simulink model "SMART_GRID_EV_as_an_Ancillary"  (R2021a)
settings: Solver=ode23tb  StartTime=0.0  StopTime=0.3  MaxStep=1e-5  RelTol=1e-3
undefined symbols (not defined in the file): DiscIntNeverNeededParam, Ion, Lithium
libraries: powerlib_extras x6, spsThreePhaseSeriesRLCBranchLib x4, spsThreePhaseVIMeasurementLib x3, spsGroundLib x2, spsBatteryLib x1, simulink x1, spsUniversalBridgeLib x1, spsThreePhaseSourceLib x1, spsThreePhaseBreakerLib x1, spspowerguiLib x1
settings Model: Creator=mo saf  LastModifiedBy=raiaj
settings SolverCC: ZeroCrossControl=DisableAll  SolverResetMethod=Robust

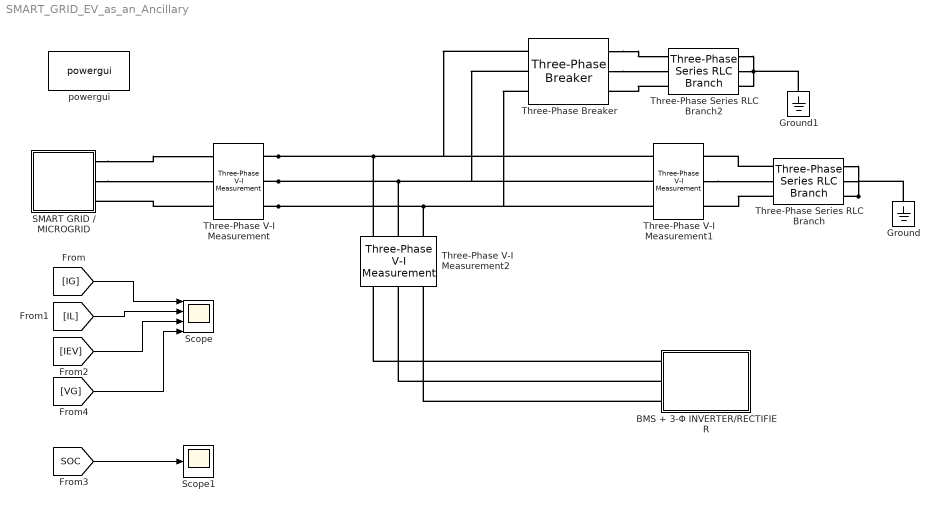
== system SMART_GRID_EV_as_an_Ancillary ==
  BMS + 3-Φ INVERTER/RECTIFIER : Subsystem
  Ground : spsGroundLib/Ground  LConnTagsString=a
  Ground1 : spsGroundLib/Ground  LConnTagsString=a
  SMART GRID / MICROGRID : Subsystem
  Scope : Scope  NumInputPorts=4
  Scope1 : Scope
  Three-Phase Series RLC Branch : spsThreePhaseSeriesRLCBranchLib/Three-Phase Series RLC Branch  LConnTagsString=A|B|C  RConnTagsString=A|B|C  BranchType=R  Resistance=20  Inductance=1e-3  Capacitance=1e-6  Measurements=None
  Three-Phase Series RLC Branch2 : spsThreePhaseSeriesRLCBranchLib/Three-Phase Series RLC Branch  LConnTagsString=A|B|C  RConnTagsString=A|B|C  BranchType=R  Resistance=6  Inductance=1e-3  Capacitance=1e-6  Measurements=None
  Three-Phase V-I Measurement : spsThreePhaseVIMeasurementLib/Three-Phase V-I Measurement  VoltageMeasurement=phase-to-ground  SetLabelV=on  LabelV=VG  Vpu=off  VpuLL=off  CurrentMeasurement=yes  SetLabelI=on  LabelI=IG  Ipu=off  Pbase=100e6  Vbase=500e3  OutputType=Complex  PhasorSimulation=off  PSBequivalent=0
  Three-Phase V-I Measurement1 : spsThreePhaseVIMeasurementLib/Three-Phase V-I Measurement  VoltageMeasurement=phase-to-ground  SetLabelV=on  LabelV=VL  Vpu=off  VpuLL=off  CurrentMeasurement=yes  SetLabelI=on  LabelI=IL  Ipu=off  Pbase=100e6  Vbase=500e3  OutputType=Complex  PhasorSimulation=off  PSBequivalent=0
  Three-Phase V-I Measurement2 : spsThreePhaseVIMeasurementLib/Three-Phase V-I Measurement  VoltageMeasurement=phase-to-ground  SetLabelV=on  LabelV=VEV  Vpu=off  VpuLL=off  CurrentMeasurement=yes  SetLabelI=on  LabelI=IEV  Ipu=off  Pbase=100e6  Vbase=500e3  OutputType=Complex  PhasorSimulation=off  PSBequivalent=0
  Three-Phase Breaker : spsThreePhaseBreakerLib/Three-Phase Breaker  InitialState=open  SwitchA=on  SwitchB=on  SwitchC=on  SwitchTimes=[0.1 9]  External=off  BreakerResistance=0.01  SnubberResistance=1e6  SnubberCapacitance=inf  Measurements=None
  powergui : spspowerguiLib/powergui  Priority=1  SimulationMode=Continuous  SampleTime=50e-6  frequency=60  Iterations=50  frequencyindice=50  Pbase=100e6  ErrMax=1e-4  UnitsV=kV  UnitsW=MW  buscounter=0  FunctionMessages=off  echomessages=off  EnableUseOfTLC=off  CurrentSourceSwitches=off  DisableSnubberDevices=off  DisableRonSwitches=off  DisableVfSwitches=off  DisplayEquations=off  AutomaticDiscreteSolvers=off  SolverType=Tustin/Backward Euler (TBE)  Interpol=off  ExternalGateDelay=off  methode=off  Ts=100  x0status=blocks  SPID=on  SwTol=0  HookPort=off  NonlinearTolerance=1e-4  nMaxIteration=100  ContinueOnMaxIteration=off  RestoreLinks=warning  ResistiveCurrentMeasurement=off  Frange=[0:2:500]  Ylog=off  Xlog=on  ShowGrid=off  save=off  variable=ZData  structure=0  ZoomFFT=off  StartTime=0.0  cycles=1  DisplayStyle=1  fundamental=60  FreqAxis=off  MaxFrequency=1000  frequencyindicesteady=1  RmsSteady=1  display=off
  wires:
  [IG] -> Scope/1
  [IEV] -> Scope/3
  [IL] -> Scope/2
  [VG] -> Scope/4
  [SOC] -> Scope1/1
  connections:
  Three-Phase V-I Measurement/RConn2 -- Three-Phase V-I Measurement2/RConn2 -- Three-Phase V-I Measurement1/LConn2 -- Three-Phase Breaker/LConn2
  Three-Phase V-I Measurement/RConn3 -- Three-Phase V-I Measurement2/RConn3 -- Three-Phase V-I Measurement1/LConn3 -- Three-Phase Breaker/LConn3
  Three-Phase Series RLC Branch2/RConn2 -- Ground1/LConn1 -- Three-Phase Series RLC Branch2/RConn1 -- Three-Phase Series RLC Branch2/RConn3
  Three-Phase Series RLC Branch/RConn3 -- Three-Phase Series RLC Branch/RConn1 -- Ground/LConn1 -- Three-Phase Series RLC Branch/RConn2
  Three-Phase V-I Measurement/RConn1 -- Three-Phase V-I Measurement1/LConn1 -- Three-Phase Breaker/LConn1 -- Three-Phase V-I Measurement2/RConn1
  Three-Phase Series RLC Branch/LConn1 -- Three-Phase V-I Measurement1/RConn1
  Three-Phase Series RLC Branch2/LConn3 -- Three-Phase Breaker/RConn3
  Three-Phase Series RLC Branch/LConn3 -- Three-Phase V-I Measurement1/RConn3
  Three-Phase V-I Measurement1/RConn2 -- Three-Phase Series RLC Branch/LConn2
  Three-Phase Breaker/RConn2 -- Three-Phase Series RLC Branch2/LConn2
  Three-Phase Breaker/RConn1 -- Three-Phase Series RLC Branch2/LConn1
  SMART GRID / MICROGRID/RConn1 -- Three-Phase V-I Measurement/LConn1
  SMART GRID / MICROGRID/RConn2 -- Three-Phase V-I Measurement/LConn2
  Three-Phase V-I Measurement/LConn3 -- SMART GRID / MICROGRID/RConn3
  BMS + 3-Φ INVERTER/RECTIFIER/LConn1 -- Three-Phase V-I Measurement2/LConn1
  BMS + 3-Φ INVERTER/RECTIFIER/LConn2 -- Three-Phase V-I Measurement2/LConn2
  BMS + 3-Φ INVERTER/RECTIFIER/LConn3 -- Three-Phase V-I Measurement2/LConn3

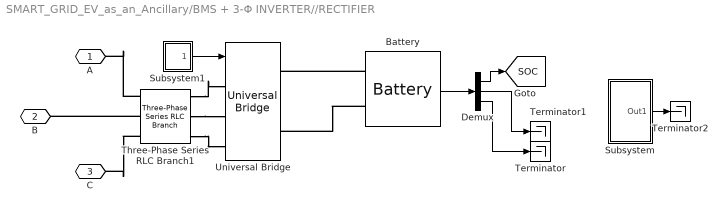
== system SMART_GRID_EV_as_an_Ancillary/BMS + 3-Φ INVERTER//RECTIFIER ==
  Battery : spsBatteryLib/Battery  BatType=Lithium-Ion  ShowTempParam=off  ThermalPreset=no  ShowAgeParam=off  NomV=700  NomQ=20  SOC=100  Batt_Tr=30  PresetModel=on  MaxQ=20  MinV=525  FullV=814.791  Dis_rate=8.6957  R=0.35  Normal_OP=18.087  expZone="[756.2701     0.9826087]"  current=[6.5 13 32.5]  Units=Time  Tci=20  NomT=20  T2=-30  MaxQ2=4.8  FullV2=7.1  Normal_OP2=5.655  expZone2="[6.58           1]"  Rca=0.6  ti=2000  Dp=0  Neq0=0  Tsim=1e6  Ta1=25  Qeol=5.4*0.9  Reol=0.013333*1.2  Char_age=[2.3478, 3]  Dis_age=[2.3478, 10]  N1=1500  N2=10500  N3=1000  N4=1400  Ta2=45  N5=950
  Demux : Demux  Outputs=3
  Subsystem : Subsystem
  Subsystem1 : Subsystem
  Terminator : Terminator
  Terminator1 : Terminator
  Terminator2 : Terminator
  Three-Phase Series RLC Branch1 : spsThreePhaseSeriesRLCBranchLib/Three-Phase Series RLC Branch  LConnTagsString=A|B|C  RConnTagsString=A|B|C  BranchType=L  Resistance=100  Inductance=2.5e-3  Capacitance=1e-6  Measurements=None
  Universal Bridge : spsUniversalBridgeLib/Universal Bridge  Arms=3  SnubberResistance=1e5  SnubberCapacitance=inf  Device=IGBT / Diodes  Ron=1e-3  Lon=0  ForwardVoltages="[  0  0  ]"  ForwardVoltage=0  GTOparameters=[ 10e-6 , 20e-6 ]  IGBTparameters=[ 1e-6 , 2e-6 ]  Measurements=None  Measurements_2=None  converterType=Rectifier
  A : PMIOPort  Side=Left
  B : PMIOPort  Port=2  Side=Left
  C : PMIOPort  Port=3  Side=Left
  tag scope: SOC=global
  wires:
  Battery/1 -> Demux/1
  Demux/2 -> Terminator1/1
  Demux/1 -> [SOC]
  Demux/3 -> Terminator/1
  Subsystem1/1(Out1) -> Universal Bridge/1
  Subsystem/1(Out1) -> Terminator2/1
  connections:
  Three-Phase Series RLC Branch1/RConn3 -- Universal Bridge/LConn3
  Battery/LConn2 -- Universal Bridge/RConn2
  Battery/LConn1 -- Universal Bridge/RConn1
  Three-Phase Series RLC Branch1/RConn2 -- Universal Bridge/LConn2
  Three-Phase Series RLC Branch1/RConn1 -- Universal Bridge/LConn1
  Three-Phase Series RLC Branch1/LConn3 -- C/RConn1
  Three-Phase Series RLC Branch1/LConn1 -- A/RConn1
  Three-Phase Series RLC Branch1/LConn2 -- B/RConn1

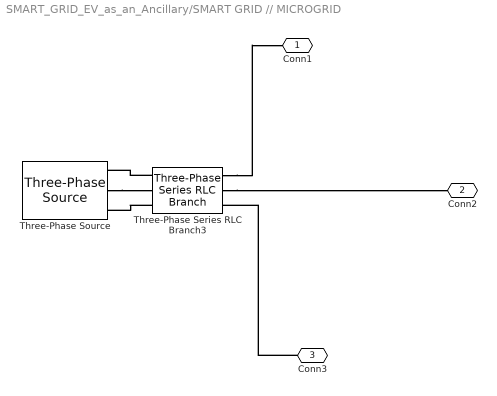
== system SMART_GRID_EV_as_an_Ancillary/SMART GRID // MICROGRID ==
  Three-Phase Series RLC Branch3 : spsThreePhaseSeriesRLCBranchLib/Three-Phase Series RLC Branch  LConnTagsString=A|B|C  RConnTagsString=A|B|C  BranchType=R  Resistance=0.1  Inductance=1e-3  Capacitance=1e-6  Measurements=None
  Three-Phase Source : spsThreePhaseSourceLib/Three-Phase Source  InternalConnection=Yg  VoltagePhases=off  Voltage=415  PhaseAngle=0  Voltage_phases=[25e3 25e3 25e3]/sqrt(3)  PhaseAngles_phases=[0 -120 +120]  Frequency=50  NonIdealSource=on  SpecifyImpedance=off  Resistance=0.8929  Inductance=16.58e-3  ShortCircuitLevel=100e6  BaseVoltage=25e3  XRratio=7  BusType=swing  Pref=10e3  Qref=0  Prefabc=[10e3, 10e3, 10e3]  Qrefabc=[0, 0, 0]  Qmin=-inf  Qmax=inf
  Conn1 : PMIOPort  Side=Right
  Conn2 : PMIOPort  Port=2  Side=Right
  Conn3 : PMIOPort  Port=3  Side=Right
  connections:
  Three-Phase Source/RConn2 -- Three-Phase Series RLC Branch3/LConn2
  Three-Phase Series RLC Branch3/LConn3 -- Three-Phase Source/RConn3
  Three-Phase Series RLC Branch3/LConn1 -- Three-Phase Source/RConn1
  Three-Phase Series RLC Branch3/RConn1 -- Conn1/RConn1
  Three-Phase Series RLC Branch3/RConn2 -- Conn2/RConn1
  Conn3/RConn1 -- Three-Phase Series RLC Branch3/RConn3

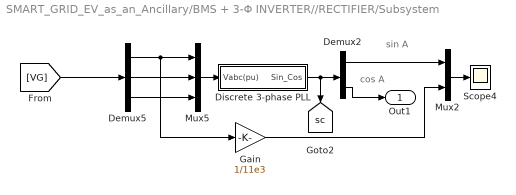
== system SMART_GRID_EV_as_an_Ancillary/BMS + 3-Φ INVERTER//RECTIFIER/Subsystem ==
  note: cos A
  note: sin A
  Demux2 : Demux  Outputs=2
  Demux5 : Demux  Outputs=3
  Discrete 3-phase PLL : Subsystem  AncestorBlock=|  DialogController=POWERSYS.PowerSysDialog  mask(Discrete 3-phase PLL){Fmin=50, Par_Init=[0 50], ParK=[ 0.02 .05 0 ], Ts=5e-6, AGC=on}
      | powerlib_extras/Discrete 
      | Control Blocks/Discrete
      | 3-phase PLL
      mask prompts: Fmin "Minimum frequency (Hz):"; Par_Init "Initial inputs:[ Phase(degrees)   Frequency(Hz) ]"; ParK "Regulator gains [ Kp  Ki  Kd ]"; Ts "Sample time:"; AGC "Enable Automatic Gain Control"
      mask help:
      | This Phase Locked Loop (PLL) system can be used  to synchronize on a set of variable frequency, three-phase sinusoidal signals. If the Automatic Gain Control is enabled, the input (phase error) of the PLL regulator is scaled according to the input signals magnitude.
      |
      | For optimal performance, the following settings are recommended:
      |   [ Kp Ki  Kd ] = [ 180  3200  1 ]
      |   "Enable Automatic Gain Control" checked
      |
      | Input 1: Vector containing the normalized three-phase signals [Va Vb Vc]
      | Output 1:  Measured frequency (Hz) = w/(2pi)
      | Output 2:  Ramp w.t varying between  0 and 2*pi,
      |      synchronized on zero crossings of the fundamental (positive-sequence) of phase A.
      | Output 3: Vector [sin(wt) cos(wt)]
      mask init:
      | Kp=ParK(1);
      | Ki=ParK(2);
      | if length(ParK)==2
      |     Kd=0;
      | else
      |     Kd=ParK(3);
      | end    
      | Phase_Init=Par_Init(1);
      | Finit=Par_Init(2);
      | power_initmask();
      settings: OpenFcn=power_openblockproxy();
      mask Display: disp('')
  Gain : Gain  Gain=1/11e3
  Mux2 : Mux  Inputs=2
  Mux5 : Mux  Inputs=3
  Scope4 : Scope
  Out1 : Outport
  tag scope: sc=global
  wires:
  Demux5/2 -> Mux5/2
  Discrete 3-phase PLL/1(Sin_Cos) -> Demux2/1, [sc]
  Demux5/1 -> Mux5/1, Gain/1
  Mux2/1 -> Scope4/1
  Gain/1 -> Mux2/2
  Demux5/3 -> Mux5/3
  Mux5/1 -> Discrete 3-phase PLL/1(Vabc(pu))
  Demux2/1 -> Mux2/1
  [VG] -> Demux5/1
  Demux2/2 -> Out1/1

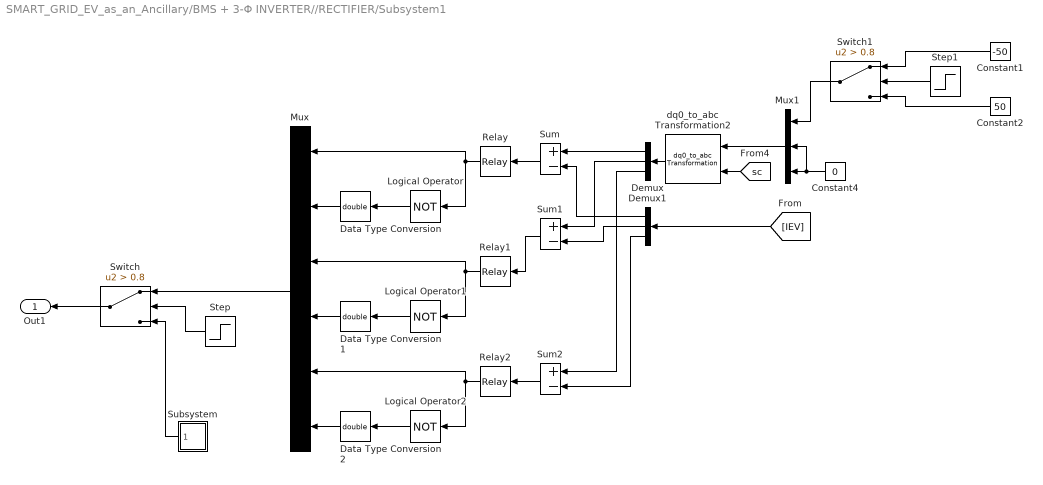
== system SMART_GRID_EV_as_an_Ancillary/BMS + 3-Φ INVERTER//RECTIFIER/Subsystem1 ==
  Constant1 : Constant  Value=-50
  Constant2 : Constant  Value=50
  Constant4 : Constant  Value=0
  Data Type Conversion : DataTypeConversion  OutDataTypeStr=double
  Data Type Conversion1 : DataTypeConversion  OutDataTypeStr=double
  Data Type Conversion2 : DataTypeConversion  OutDataTypeStr=double
  Demux : Demux  Outputs=3
  Demux1 : Demux  Outputs=3
  Logical Operator : Logic  Operator=NOT  AllPortsSameDT=off  OutDataTypeStr=boolean
  Logical Operator1 : Logic  Operator=NOT  AllPortsSameDT=off  OutDataTypeStr=boolean
  Logical Operator2 : Logic  Operator=NOT  AllPortsSameDT=off  OutDataTypeStr=boolean
  Mux : Mux  Inputs=6
  Mux1 : Mux  Inputs=3
  Relay : Relay  OnSwitchValue=0.05  OffSwitchValue=-0.05
  Relay1 : Relay  OnSwitchValue=0.05  OffSwitchValue=-0.05
  Relay2 : Relay  OnSwitchValue=0.05  OffSwitchValue=-0.05
  Step : Step  Time=0.2  SampleTime=0
  Step1 : Step  Time=9  SampleTime=0
  Subsystem : Subsystem
  Sum : Sum  Inputs=+-
  Sum1 : Sum  Inputs=+-
  Sum2 : Sum  Inputs=+-
  Switch : Switch  Criteria=u2 > Threshold  Threshold=0.8
  Switch1 : Switch  Criteria=u2 > Threshold  Threshold=0.8
  dq0_to_abc Transformation2 : powerlib_extras/Measurements/dq0_to_abc Transformation
      settings: SourceProductBaseCode=PS
  Out1 : Outport
  wires:
  Relay1/1 -> Mux/3, Logical Operator1/1
  Demux1/2 -> Sum1/2
  Mux1/1 -> dq0_to_abc Transformation2/1
  Constant4/1 -> Mux1/2, Mux1/3
  [sc] -> dq0_to_abc Transformation2/2
  Sum/1 -> Relay/1
  Demux/2 -> Sum1/1
  Relay2/1 -> Mux/5, Logical Operator2/1
  Demux/3 -> Sum2/1
  Data Type Conversion1/1 -> Mux/4
  Relay/1 -> Logical Operator/1, Mux/1
  Logical Operator1/1 -> Data Type Conversion1/1
  Sum1/1 -> Relay1/1
  Data Type Conversion/1 -> Mux/2
  Data Type Conversion2/1 -> Mux/6
  dq0_to_abc Transformation2/1 -> Demux/1
  Demux1/3 -> Sum2/2
  [IEV] -> Demux1/1
  Demux1/1 -> Sum/2
  Sum2/1 -> Relay2/1
  Demux/1 -> Sum/1
  Logical Operator/1 -> Data Type Conversion/1
  Logical Operator2/1 -> Data Type Conversion2/1
  Switch/1 -> Out1/1
  Subsystem/1(Out1) -> Switch/3
  Mux/1 -> Switch/1
  Step/1 -> Switch/2
  Step1/1 -> Switch1/2
  Switch1/1 -> Mux1/1
  Constant1/1 -> Switch1/1
  Constant2/1 -> Switch1/3

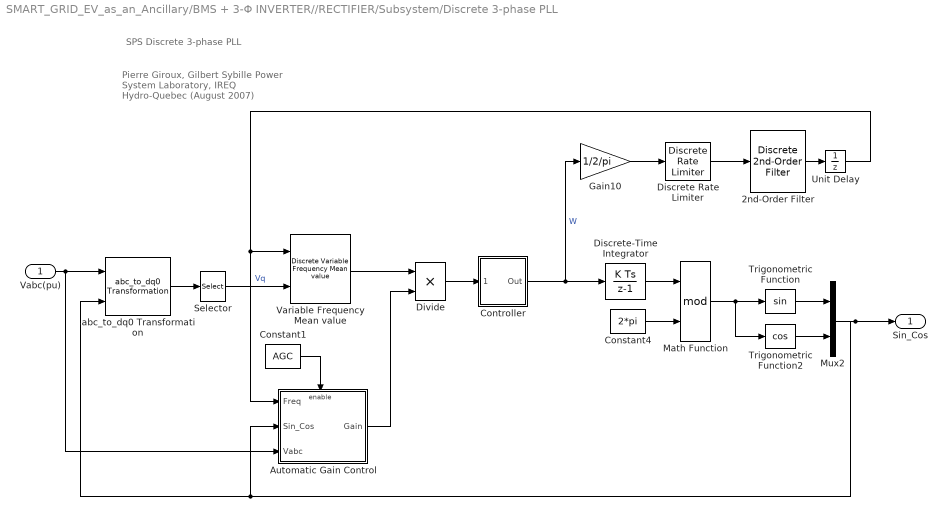
== system SMART_GRID_EV_as_an_Ancillary/BMS + 3-Φ INVERTER//RECTIFIER/Subsystem/Discrete 3-phase PLL ==
  note: SPS Discrete 3-phase PLL
  note: Pierre Giroux, Gilbert Sybille
      | Power System Laboratory, IREQ
      | Hydro-Quebec
      | (August 2007)
  Vabc(pu) : Inport  PortDimensions=3
  2nd-Order Filter : powerlib_extras/Discrete  Control Blocks/Discrete  2nd-Order Filter  FilterType=Lowpass  Fo=25  Zeta=0.707  Ts=Ts  Initialize=on  Vac_Init=[0 0 Finit]  Vdc_Init=Finit  PlotResponse=off  param1=[1 500 0.1]
      settings: SourceProductBaseCode=PS
  Automatic Gain Control : Subsystem  TreatAsAtomicUnit=on
  Constant1 : Constant  Value=AGC
  Constant4 : Constant  Value=2*pi
  Controller : Subsystem  mask(Discrete PID Controller){Kp=Kp, Ki=Ki, Kd=Kd, Par_Limits=[10000 0], Init=2*pi*Finit, Ts=Ts}
      mask prompts: Kp "Proportional gain (Kp):"; Ki "Integral gain (Ki):"; Kd "Derivative gain (Kd):"; Par_Limits "Output limits: [ Upper   Lower ]"; Init "Output initial value:"; Ts "Sample time:"
      mask help: This block implements a discrete PID controller.
      mask init:
      | UpperLimit=Par_Limits(1);
      | LowerLimit=Par_Limits(2);
      | power_initmask();
      settings: OpenFcn=power_openblockproxy();
      mask Display: disp('PID');
  Discrete Rate Limiter : powerlib_extras/Discrete  Control Blocks/Discrete Rate Limiter  R=12  F=-12  Vinit=Finit  Ts=Ts
      settings: SourceProductBaseCode=PS
  Discrete-Time Integrator : DiscreteIntegrator  InitialCondition=Phase_Init*pi/180  SampleTime=Ts  ICPrevOutput=DiscIntNeverNeededParam  ICPrevScaledInput=DiscIntNeverNeededParam
  Divide : Product
  Gain10 : Gain  Gain=1/2/pi  SaturateOnIntegerOverflow=on  OutDataTypeStr=Inherit: Same as input  ParamDataTypeStr=Inherit: Same as input
  Math Function : Math  Operator=mod  SignedPower=on  SaturateOnIntegerOverflow=on
  Mux2 : Mux  Inputs=2
  Selector : Selector  InputPortWidth=3  IndexOptions=Index vector (dialog)  Indices=2  OutputSizes=1
  Trigonometric Function : Trigonometry
  Trigonometric Function2 : Trigonometry  Operator=cos
  Unit Delay : UnitDelay  InitialCondition=Finit  SampleTime=Ts  HasFrameUpgradeWarning=on
  Variable Frequency Mean value : powerlib_extras/Discrete Measurements/Discrete Variable Frequency Mean value  Finit=Finit  Fmin=Fmin  Vinit=0  Ts=Ts
      settings: SourceProductBaseCode=PS
  abc_to_dq0 Transformation : powerlib_extras/Measurements/abc_to_dq0 Transformation
      settings: SourceProductBaseCode=PS
  Sin_Cos : Outport
  wires:
  Constant1/1 -> Automatic Gain Control/Enable
  Divide/1 -> Controller/1(Error)
  Automatic Gain Control/1(Gain) -> Divide/2
  Variable Frequency Mean value/1 -> Divide/1
  Controller/1(Out) -> Gain10/1, Discrete-Time Integrator/1  "W"
  Vabc(pu)/1 -> Automatic Gain Control/3(Vabc), abc_to_dq0 Transformation/1
  abc_to_dq0 Transformation/1 -> Selector/1
  Constant4/1 -> Math Function/2
  Discrete-Time Integrator/1 -> Math Function/1
  Math Function/1 -> Trigonometric Function2/1, Trigonometric Function/1
  Trigonometric Function/1 -> Mux2/1
  Trigonometric Function2/1 -> Mux2/2
  Mux2/1 -> Automatic Gain Control/2(Sin_Cos), abc_to_dq0 Transformation/2, Sin_Cos/1
  Gain10/1 -> Discrete Rate Limiter/1
  Discrete Rate Limiter/1 -> 2nd-Order Filter/1
  Unit Delay/1 -> Automatic Gain Control/1(Freq), Variable Frequency Mean value/1
  2nd-Order Filter/1 -> Unit Delay/1
  Selector/1 -> Variable Frequency Mean value/2  "Vq"

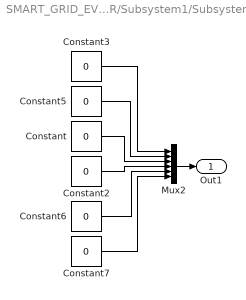
== system SMART_GRID_EV_as_an_Ancillary/BMS + 3-Φ INVERTER//RECTIFIER/Subsystem1/Subsystem ==
  Constant{,2..3,5..7} (6 alike) : Constant  Value=0
  Mux2 : Mux  Inputs=6
  Out1 : Outport
  wires:
  Constant3/1 -> Mux2/1
  Constant5/1 -> Mux2/2
  Constant6/1 -> Mux2/5
  Constant2/1 -> Mux2/4
  Constant7/1 -> Mux2/6
  Constant/1 -> Mux2/3
  Mux2/1 -> Out1/1

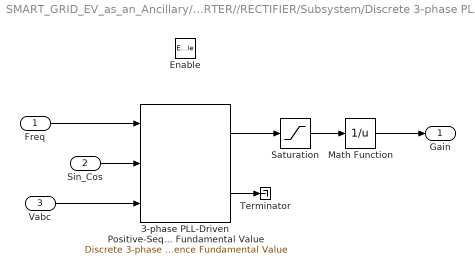
== system SMART_GRID_EV_as_an_Ancillary/BMS + 3-Φ INVERTER//RECTIFIER/Subsystem/Discrete 3-phase PLL/Automatic Gain Control ==
  Freq : Inport
  Sin_Cos : Inport  Port=2
  Vabc : Inport  Port=3
  Enable : EnablePort  PropagateVarSize=During execution
  3-phase PLL-Driven Positive-Sequence Fundamental Value : powerlib_extras/Discrete Measurements/Discrete 3-phase PLL-Driven Positive-Sequence Fundamental Value  Finit=Finit  Fmin=Fmin  Par_Init=[1 0]  Ts=Ts
      settings: SourceProductBaseCode=PS
  Math Function : Math  Operator=reciprocal  SignedPower=on  SaturateOnIntegerOverflow=on
  Saturation : Saturate  UpperLimit=2  LowerLimit=0.01
  Terminator : Terminator
  Gain : Outport  InitialOutput=[1]
  wires:
  Math Function/1 -> Gain/1
  Vabc/1 -> 3-phase PLL-Driven Positive-Sequence Fundamental Value/3
  Sin_Cos/1 -> 3-phase PLL-Driven Positive-Sequence Fundamental Value/2
  Freq/1 -> 3-phase PLL-Driven Positive-Sequence Fundamental Value/1
  3-phase PLL-Driven Positive-Sequence Fundamental Value/1 -> Saturation/1
  Saturation/1 -> Math Function/1
  3-phase PLL-Driven Positive-Sequence Fundamental Value/2 -> Terminator/1

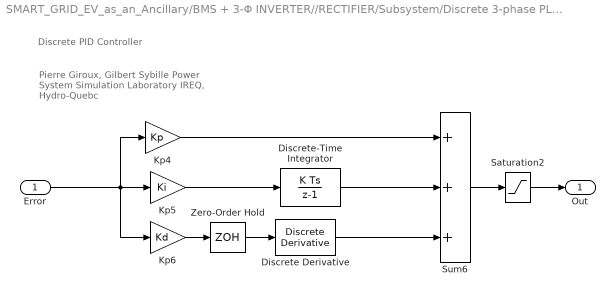
== system SMART_GRID_EV_as_an_Ancillary/BMS + 3-Φ INVERTER//RECTIFIER/Subsystem/Discrete 3-phase PLL/Controller ==
  note: Discrete PID Controller
  note: Pierre Giroux, Gilbert Sybille
      | Power System Simulation Laboratory
      | IREQ, Hydro-Quebc
  Error : Inport
  Discrete Derivative : simulink/Discrete/Discrete Derivative  gainval=1.0  ICPrevScaledInput=0.0  OutMin=[]  OutMax=[]  OutDataType=fixdt(1, 16)  OutScaling=2^-10  DoSatur=off
  Discrete-Time Integrator : DiscreteIntegrator  InitialCondition=Init  SampleTime=Ts  LimitOutput=on  UpperSaturationLimit=UpperLimit  LowerSaturationLimit=LowerLimit  ICPrevOutput=DiscIntNeverNeededParam  ICPrevScaledInput=DiscIntNeverNeededParam
  Kp4 : Gain  Gain=Kp  SaturateOnIntegerOverflow=on  OutDataTypeStr=Inherit: Same as input  ParamDataTypeStr=Inherit: Same as input
  Kp5 : Gain  Gain=Ki  SaturateOnIntegerOverflow=on  OutDataTypeStr=Inherit: Same as input  ParamDataTypeStr=Inherit: Same as input
  Kp6 : Gain  Gain=Kd  SaturateOnIntegerOverflow=on  OutDataTypeStr=Inherit: Same as input  ParamDataTypeStr=Inherit: Same as input
  Saturation2 : Saturate  UpperLimit=UpperLimit  LowerLimit=LowerLimit
  Sum6 : Sum  Inputs=+++  InputSameDT=on  SaturateOnIntegerOverflow=on  OutDataTypeStr=Inherit: Same as first input
  Zero-Order Hold : ZeroOrderHold  SampleTime=Ts
  Out : Outport  InitialOutput=0
  wires:
  Zero-Order Hold/1 -> Discrete Derivative/1
  Saturation2/1 -> Out/1
  Discrete Derivative/1 -> Sum6/3
  Discrete-Time Integrator/1 -> Sum6/2
  Kp4/1 -> Sum6/1
  Kp6/1 -> Zero-Order Hold/1
  Kp5/1 -> Discrete-Time Integrator/1
  Sum6/1 -> Saturation2/1
  Error/1 -> Kp6/1, Kp5/1, Kp4/1
